simulink model "Punto_1"  (R2025b)
settings: Solver=VariableStepAuto  StartTime=0.0  StopTime=10  RelTol=1e-3
values from neighbouring files (symbols this model uses):
  kd = 48.616    [Punto_1_Cod.m]
  ki = 39.46    [Punto_1_Cod.m]
  kp = -8405.61    [Punto_1_Cod.m]    (also in Punto_3_Cod.m = 0.114)
  q0 = (kd/T) + kp + (ki*T)    (= -8302.70879163)    [Punto_1_Cod.m]    (also in Punto_3_Cod.m = 0.62989408)
  q1 = - (2*kd/T) - kp    (= 8356.70054326)    [Punto_1_Cod.m]    (also in Punto_3_Cod.m = -1.08976)
  q2 = kd/T    (= 24.4547283702)    [Punto_1_Cod.m]    (also in Punto_3_Cod.m = 0.628)
  T = 1.988    [Punto_1_Cod.m]    (also in Punto_3_Cod.m = 52)
undefined symbols (not defined in the file or in its folder): dspblkCoreblockFVToolHelper, gcbh
settings Model: Creator=Andres Felipe  LastModifiedBy=Andres Felipe

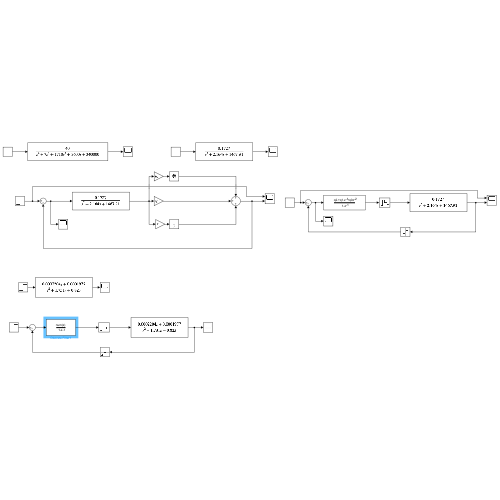
[thumbnail: Simulink's stored preview of the top-level diagram]
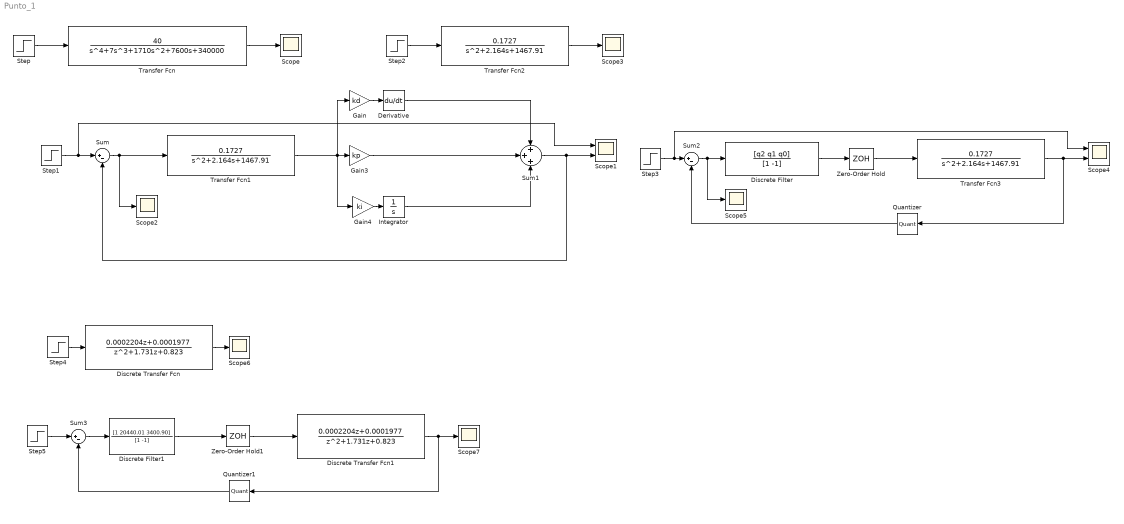
== system Punto_1 ==
  Derivative : Derivative
  Discrete Transfer Fcn : DiscreteTransferFcn  Numerator=[0.0002204 0.0001977]  Denominator=[1 1.731 0.823]
  Discrete Transfer Fcn1 : DiscreteTransferFcn  Numerator=[0.0002204 0.0001977]  Denominator=[1 1.731 0.823]
  Discrete Filter : DiscreteFilter  Numerator=[q2 q1 q0]  Denominator=[1 -1]  FilterStructure=Direct form II transposed
  Discrete Filter1 : DiscreteFilter  LoadFcn=dspblkCoreblockFVToolHelper(gcbh,'load');  Numerator=[1 20440.01 3400.90]  Denominator=[1 -1]
      settings: CopyFcn=dspblkCoreblockFVToolHelper(gcbh,'copy');  DeleteFcn=dspblkCoreblockFVToolHelper(gcbh,'close');  ModelCloseFcn=dspblkCoreblockFVToolHelper(gcbh,'close');  PreSaveFcn=dspblkCoreblockFVToolHelper(gcbh,'presave');  PostSaveFcn=dspblkCoreblockFVToolHelper(gcbh,'postsave');  CloseFcn=dspblkCoreblockFVToolHelper(gcbh,'close');
  Gain : Gain  Gain=kd
  Gain3 : Gain  Gain=kp
  Gain4 : Gain  Gain=ki
  Integrator : Integrator
  Quantizer : Quantizer  QuantizationInterval=3.3/1023
  Quantizer1 : Quantizer  QuantizationInterval=3.3/1023
  Scope{,2..3,5..7} (6 alike) : Scope
      Scope settings: ActiveDisplayYMinimum=-2.60485540886865E-5  ActiveDisplayYMaximum=0.00023443698679817855
      Scope2 settings: ActiveDisplayYMinimum=-8.3278479816761841  ActiveDisplayYMaximum=77.603658213763879  DataLoggingVariableName=ScopeData2
      Scope3 settings: ActiveDisplayYMinimum=-2.7806178227628586E-5  ActiveDisplayYMaximum=0.00025025560404865735  DataLoggingVariableName=ScopeData3
      Scope5 settings: ActiveDisplayYMinimum=-1  ActiveDisplayYMaximum=1  DataLoggingVariableName=ScopeData5
      Scope6 settings: ActiveDisplayYMinimum=-1  ActiveDisplayYMaximum=1  DataLoggingVariableName=ScopeData6
      Scope7 settings: ActiveDisplayYMinimum=-2.7549999999999992E-5  ActiveDisplayYMaximum=0.00024795  DataLoggingVariableName=ScopeData7
  Scope1 : Scope  NumInputPorts=2
      settings: ActiveDisplayYMinimum=-76.636821043497363  ActiveDisplayYMaximum=9.6263134492774824
  Scope4 : Scope  NumInputPorts=2
      settings: ActiveDisplayYMinimum=-0.94715877149171446  ActiveDisplayYMaximum=2.1611515001786903  DataLoggingVariableName=ScopeData4
  Step{,1..5} (6 alike) : Step  Time=0  SampleTime=0
  Sum : Sum  Inputs=|+-
  Sum1 : Sum  Inputs=+++
  Sum2 : Sum  Inputs=|+-
  Sum3 : Sum  Inputs=|+-
  Transfer Fcn : TransferFcn  Numerator=[40]  Denominator=[1 7 1710 7600 340000]
  Transfer Fcn1 : TransferFcn  Numerator=[0.1727]  Denominator=[1 2.164 1467.91]
  Transfer Fcn2 : TransferFcn  Numerator=[0.1727]  Denominator=[1 2.164 1467.91]
  Transfer Fcn3 : TransferFcn  Numerator=[0.1727]  Denominator=[1 2.164 1467.91]
  Zero-Order Hold : ZeroOrderHold  SampleTime=T
  Zero-Order Hold1 : ZeroOrderHold  SampleTime=0.09
  wires:
  Transfer Fcn/1 -> Scope/1
  Step/1 -> Transfer Fcn/1
  Transfer Fcn2/1 -> Scope3/1
  Step2/1 -> Transfer Fcn2/1
  Transfer Fcn1/1 -> Gain/1, Gain4/1, Gain3/1
  Step1/1 -> Sum/1, Scope1/1
  Gain/1 -> Derivative/1
  Sum/1 -> Transfer Fcn1/1, Scope2/1
  Derivative/1 -> Sum1/1
  Integrator/1 -> Sum1/3
  Gain3/1 -> Sum1/2
  Sum1/1 -> Sum/2, Scope1/2
  Gain4/1 -> Integrator/1
  Transfer Fcn3/1 -> Quantizer/1, Scope4/2
  Step3/1 -> Scope4/1, Sum2/1
  Sum2/1 -> Scope5/1, Discrete Filter/1
  Discrete Filter/1 -> Zero-Order Hold/1
  Zero-Order Hold/1 -> Transfer Fcn3/1
  Quantizer/1 -> Sum2/2
  Step4/1 -> Discrete Transfer Fcn/1
  Discrete Transfer Fcn/1 -> Scope6/1
  Sum3/1 -> Discrete Filter1/1
  Step5/1 -> Sum3/1
  Discrete Transfer Fcn1/1 -> Quantizer1/1, Scope7/1
  Zero-Order Hold1/1 -> Discrete Transfer Fcn1/1
  Discrete Filter1/1 -> Zero-Order Hold1/1
  Quantizer1/1 -> Sum3/2
